simulink model "control_assi2"  (R2021a)
settings: Solver=VariableStepAuto  StartTime=0.0  StopTime=30  RelTol=1e-3
settings Model: Creator=User  LastModifiedBy=User

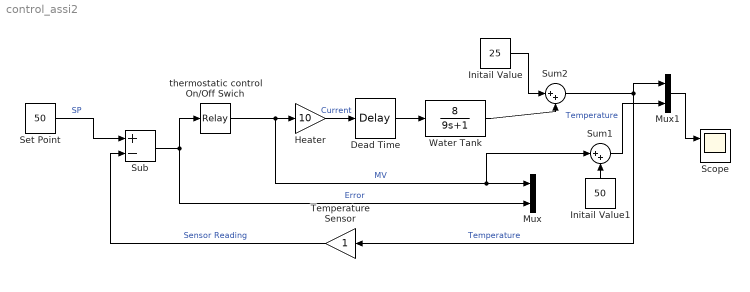
== system control_assi2 ==
  Dead Time : TransportDelay  DelayTime=0.5
  Heater : Gain  Gain=10
  Initail Value : Constant  Value=25
  Initail Value1 : Constant  Value=50
  Mux : Mux  Inputs=2
  Mux1 : Mux  Inputs=2
  Scope : Scope  NumInputPorts=2
  Set Point : Constant  Value=50
  Sub : Sum  Inputs=+-
  Sum1 : Sum  Inputs=|++
  Sum2 : Sum  Inputs=|++
  Temperature Sensor : Gain
  Water Tank : TransferFcn  Numerator=[8]  Denominator=[9 1]
  thermostatic control On/Off Swich : Relay  OnSwitchValue=2  OffSwitchValue=-2
  wires:
  Temperature Sensor/1 -> Sub/2  "Sensor Reading"
  Set Point/1 -> Sub/1  "SP"
  Sub/1 -> thermostatic control On/Off Swich/1, Mux/2  "Error"
  Sum2/1 -> Mux1/1, Temperature Sensor/1  "Temperature"
  Water Tank/1 -> Sum2/2
  Initail Value/1 -> Sum2/1
  Heater/1 -> Dead Time/1  "Current"
  Dead Time/1 -> Water Tank/1
  thermostatic control On/Off Swich/1 -> Sum1/1, Mux/1, Heater/1  "MV"
  Mux1/1 -> Scope/1
  Initail Value1/1 -> Sum1/2
  Sum1/1 -> Mux1/2  "Temperature"
